simulink library "EngineSystemSubmodel"  (R2014b)
settings: Solver=ode45  StartTime=0.0  StopTime=10.0  FixedStep=1e-4  RelTol=1e-3
values from neighbouring files (symbols this model uses):
  D_turb_wheel = TC.TC_map.turb.D_wheel    [init_MVM.m]
  delta = 2    [Init8RTFLEX68D.m]    (also in Untitled2.m = fcn(p); fcn.m = zeros(size(p)))
  eta_turb_max = TC.TC_map.turb.eff_max    [init_MVM.m]
  flow_coeff_turb = [-1.585326540339;-4.823836967181;1.5853156139822]    [Init8RTFLEX68D.m]    (also in init_MVM.m = TC.TC_map.turb.flow_fit_coeff)
  fs = 0.0683    [Init8RTFLEX68D.m]    (also in NOxProcessGUI.m = varargin{2}; initHybrid.m; initMV.m; init_MVM.m = 0.0682925799315)
  genset = generators(1)    [runTempCyl4S.m]
  J_tc = TC.SAE_map_comp.inertia    [init_MVM.m]
  kai = 1.7    [Init8RTFLEX68D.m]
  Kb = 1*ones(engines,1)    [initHybrid.m]    (also in initMV.m; init_MVM.m = 1; init_ele.m = 1)
  Kd = 20*ones(engines,1)    [initHybrid.m]    (also in initMV.m; init_MVM.m = 10; init_ele.m = 20)
  Ki = 20*ones(engines,1)    [initHybrid.m]    (also in initMV.m; init_MVM.m = 10; init_ele.m = 20)
  Kp = 20*ones(engines,1)    [initHybrid.m]    (also in initMV.m; init_MVM.m = 10; init_ele.m = 20)
  Load_amp = x(4) + xRef(i)    [GetErrGensetResp.m]    (also in runsimulation.m = 0.55; runsimulationRecovery.m = InitialLoad(jj) + LoadStep(ii))
  Load_bias = x(4)    [GetErrGensetResp.m]    (also in runsimulation.m = 0.15; runsimulationRecovery.m = InitialLoad(jj))
  Load_index = 1    [GetErrGensetResp.m]    (also in runsimulation.m; runsimulationRecovery.m)
  N = x*noMol    [NOxProcessGUI.m]    (also in initHybrid.m = .1*ones(engines,1); initMV.m = .1*ones(engines,1); init_ele.m = 0.1)
  omegat0 = RPM_TC_initial/30*pi    [init_MVM.m]
  Start_time = 50    [GetErrGensetResp.m]    (also in runsimulation.m; runsimulationRecovery.m)
  T_load = 1    [GetErrGensetResp.m]    (also in runsimulation.m; runsimulationRecovery.m)
  T_ref_turb = TC.TC_map.turb.T_ref    [init_MVM.m]
  u0 = 0.2    [init_MVM.m]
  Uc_opt = TC.TC_map.turb.Uc_opt    [init_MVM.m]
  uMax = 1.5*ones(engines,1)    [initHybrid.m]    (also in initMV.m; init_MVM.m = 1.1; init_ele.m = 1.1)
  uMin = 0*ones(engines,1)    [initHybrid.m]    (also in initMV.m; init_MVM.m = 0.1; init_ele.m = 0.1)
undefined symbols (not defined in the file or in its folder): CAIPO, control, CV, cyl, eng, engSCont, omega0, rhoG0, Td, Ti, turbo, u_max, volDisp, vSCont, vSDes
undefined symbols (not defined in the file): comp_eff_map, comp_flow_map, n288_rep, npr, nsp, pr_rep, vComp
libraries: EngineSystemSubmodel x167, simulink x2
(part 1 of 5)
settings Model: Creator=yum  LastModifiedBy=yum

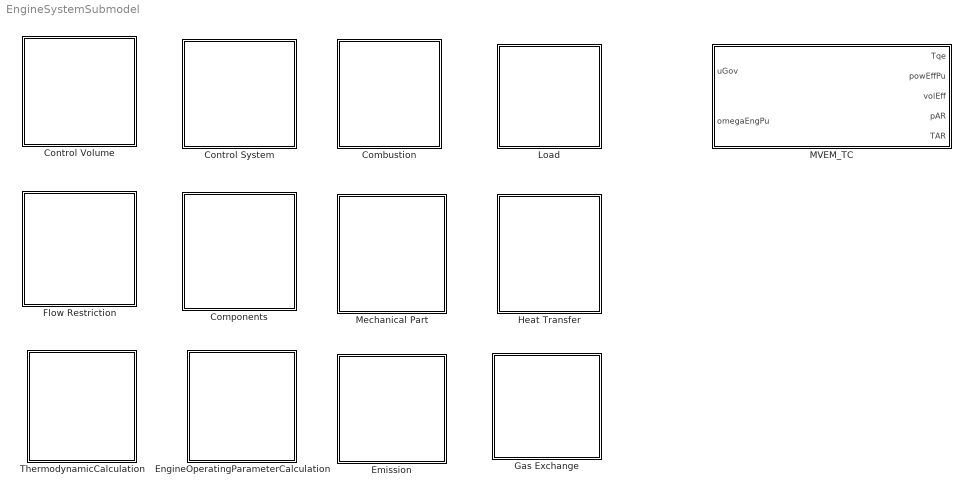
== system EngineSystemSubmodel ==
  Combustion : Subsystem
  Components : Subsystem
  Control System : Subsystem
  Control Volume : Subsystem
  Emission : Subsystem
  EngineOperatingParameterCalculation : Subsystem
  Flow Restriction : Subsystem
  Gas Exchange : Subsystem
  Heat Transfer : Subsystem
  Load : Subsystem
  MVEM_TC : Subsystem  mask{eng=genset.eng}
      mask prompts: eng "Genset parameters"
  Mechanical Part : Subsystem
  ThermodynamicCalculation : Subsystem

== system EngineSystemSubmodel/Combustion ==
  ROHR : Subsystem
  ROHRBus : Subsystem

== system EngineSystemSubmodel/Components ==
  ControlValve : Subsystem  mask{valveOpRef=0, KvRef=0}
      mask prompts: valveOpRef "Valve opening reference array (0~1)"; KvRef "Valve coefficient reference array (Kv) [m3/h]"
  EngCylinder2Stroke : Subsystem  mask{cylPar=eng.cyl, cylNo=1, cyl=0}
      mask prompts: cylPar "Cylinder parameters (struct)"; cylNo "Cylinder number"; cyl "Cylinder parameters"
      mask init:
      | cyl=cylPar(cylNo);
  EngCylinder2StrokeBus : Subsystem  mask{cylPar=eng.cyl, cylNo=1, cyl=0}
      mask prompts: cylPar "Engine Cylinder Parameters  (struct)"; cylNo "Cylinder number"; cyl "Engine Cylinder Parameters"
      mask init:
      | cyl=cylPar(cylNo);
  EngCylinder2StrokeBusConv : Subsystem  mask{cylPar=eng.cyl, cylNo=1, cyl=0}
      mask prompts: cylPar "Engine Cylinder Parameters  (struct)"; cylNo "Cylinder number"; cyl "Engine Cylinder Parameters"
      mask init:
      | cyl=cylPar(cylNo);
  EngCylinder2StrokeBusSSTune : Subsystem  mask{cylPar=eng.cyl, cylNo=1, cyl=eng.cyl}
      mask prompts: cylPar "Engine Cylinder Parameters  (struct)"; cylNo "Cylinder number"; cyl "Engine Cylinder Parameters"
      mask init:
      | cyl=cylPar(cylNo);
  EngCylinder2StrokeConv : Subsystem  mask{cylPar=eng.cyl, cylNo=1, cyl=0}
      mask prompts: cylPar "Cylinder Parameter (Struct)"; cylNo "Cylinder number"; cyl "Cylinder Parameter"
      mask init:
      | cyl = cylPar(cylNo);
  EngCylinder2StrokeSSTune : Subsystem  mask{cylPar=eng.cyl, cylNo=2, cyl=eng.cyl}
      mask prompts: cylPar "Cylinder parameters (struct)"; cylNo "Cylinder number"; cyl "Cylinder parameters"
      mask init:
      | cyl=cylPar(cylNo);
  EngCylinder2StrokeSSTune_ExtendedOutput : Subsystem  mask{cylPar=eng.cyl, cylNo=1, cyl=eng.cyl}
      mask prompts: cylPar "Cylinder Parameter (struct)"; cylNo "Cylinder number"; cyl "Cylinder Parameter"
      mask init:
      | cyl = cylPar(cylNo);
  EngCylinder2Stroke_ExtendedOutput : Subsystem  mask{cylPar=eng.cyl, cylNo=1, cyl=eng.cyl}
      mask prompts: cylPar "Cylinder Parameter (struct)"; cylNo "Cylinder number"; cyl "Cylinder Parameter"
      mask init:
      | cyl = cylPar(cylNo);
  EngCylinder2Zone2StrokeBusConv_Do Not Use : Subsystem  mask{cylPar=eng.cyl, cylNo=1, cyl=0}
      mask prompts: cylPar "Engine Cylinder Parameters  (struct)"; cylNo "Cylinder number"; cyl "Engine Cylinder Parameters"
      mask init:
      | cyl=cylPar(cylNo);
  EngCylinder2Zone2StrokeBus_Do Not Use : Subsystem  mask{cylPar=eng.cyl, cylNo=1, cyl=0}
      mask prompts: cylPar "Engine Cylinder Parameters  (struct)"; cylNo "Cylinder number"; cyl "Engine Cylinder Parameters"
      mask init:
      | cyl=cylPar(cylNo);
  EngCylinder4Stroke : Subsystem  mask{cyl=eng.cyl, cylNo=1}
      mask prompts: cyl "Engine Cylinder Parameters  (struct)"; cylNo "Cylinder number"
  EngineCylinderBlock2Stroke : Subsystem
  EngineCylinderBlock2StrokeBus : Subsystem
  EngineCylinderBlock2StrokeBusConv : Subsystem
  EngineCylinderBlock2StrokeBusSSTune : Subsystem
  EngineCylinderBlock2StrokeSSTune : Subsystem
  EngineCylinderBlock4StrokeBus : Subsystem
  ExhValve : Subsystem
  ExhValveBus : Subsystem
  ExhValveBusAEffAdjust : Subsystem
  InCylinderMV : Subsystem  mask{fs=0, Vd=0, LHV=0, Pe_nom=0, SFC=0, vol_eff_coeff1=0, vol_eff_coeff2=0, T_pe=0, nstroke=0, m_f_cyc_max=0, C1=0, p_a_inf=0, Pe0=0}
      mask prompts: fs "Stoichiometric fuel-air ratio"; Vd "Displacement volume (m3)"; LHV "Lower heating value of the fuel (J/kg)"; Pe_nom "Rated shaft power (W)"; SFC "Quadratic SFC curve coefficient (3x1)"; vol_eff_coeff1 "Volumetric efficiency coefficient for higher inlet pressure"; vol_eff_coeff2 "Volumetric efficiency coefficient for lower inlet pressure"; T_pe "Time constant for the torque development"; nstroke "Number of stroke"; m_f_cyc_max "Maximum amount of fuel injected per cycle (kg)"; C1 "Heat loss coefficient"; p_a_inf "Upper pressure limit for volumetric efficiency model 1 [bar]"; Pe0 "Initial power"
      mask TypeOptions fs: S-Function/fs
      mask TypeOptions Vd: S-Function/Vd
      mask TypeOptions LHV: S-Function/LHV
      mask TypeOptions Pe_nom: S-Function/Pe_nom
      mask TypeOptions SFC: S-Function/SFC
      mask TypeOptions vol_eff_coeff1: S-Function/vol_eff_coeff1
      mask TypeOptions vol_eff_coeff2: S-Function/vol_eff_coeff2
      mask TypeOptions T_pe: S-Function/T_pe
      mask TypeOptions nstroke: S-Function/nstroke
      mask TypeOptions m_f_cyc_max: S-Function/m_f_cyc_max
      mask TypeOptions C1: S-Function/C1
      mask TypeOptions p_a_inf: S-Function/p_a_inf
      mask TypeOptions Pe0: S-Function/Pe0
  InCylinderMVBus : Subsystem  mask{cyl=eng.cyl}
  IntakePort : Subsystem
  IntakePortBus : Subsystem
  IntakeValve : Subsystem
  IntakeValveBus : Subsystem
  IntakeValveBusAEffAdjust : Subsystem
  Turbocharger : Subsystem  mask{turbo=turbo}
      mask prompts: turbo "Turbocharger parameters struct"
  TurbochargerFullModel : Subsystem  mask{turbo=eng.turbo}
      mask prompts: turbo "Turbocharger parameters"
  TurbochargerMV : Subsystem  mask{fs=fs, J_tc=J_tc, omegat0=omegat0, comp_flow_map=comp_flow_map, comp_eff_map=comp_eff_map, pr_rep=pr_rep, n_288_rep=n288_rep, npr=npr, nsp=nsp, flow_coeff_turb=flow_coeff_turb, D_wheel_turb=D_turb_wheel, Uc_opt=Uc_opt, eta_turb_max=eta_turb_max, T_ref=T_ref_turb}
      mask prompts: fs "Stoichiometric fuel-air ratio"; J_tc "Mass moment of inertia of a rotor"; omegat0 "Initial rotor speed"; comp_flow_map "Compressor map for corrected flow"; comp_eff_map "Compressor map for efficiency"; pr_rep "Pressure ratio arry for look-up in compressor map"; n_288_rep "Corrected speed array for look-up in compressor map"; npr "Length of pressure ratio array for look-up in compressor map"; nsp "Length of corrected speed array for look-up in compressor map"; flow_coeff_turb "Flow coefficient for turbine model"; D_wheel_turb "Turbine wheel diameter"; Uc_opt "Optimal blade speed ratio"; eta_turb_max "Maximum efficiency"; T_ref "Reference temperature for turbine flow"
  WasteGate : Subsystem

== system EngineSystemSubmodel/Control System ==
  ECSParamId : Subsystem  mask{control=eng.control}
      mask prompts: control "Control Parameters"
  ECSTrans : Subsystem  mask{control=eng.control}
      mask prompts: control "Engine Control Parameters"
  ECSTrans1 : Subsystem  mask{control=eng.control}
      mask prompts: control "Engine Control Parameters"
  ECSTransSmokeLim : Subsystem  mask{control=eng.control}
      mask prompts: control "Engine Control Parameters"
  Governor : Subsystem
  Governor_SpeedControl : Subsystem  mask{Kp=Kp, Kd=Kd, N=0, Ki=Ki, Kb=Kb, omega0=omega0, u_min=u_max, u_max=u_max, u0=u0}
      mask prompts: Kp "Proportional gain"; Kd "Differential gain"; N "Dirty derivative gain"; Ki "Integral gain"; Kb "Back-calculation gain"; omega0 "Initial engine speed [pu]"; u_min "Minimum governor output"; u_max "Maximum governor output"; u0 "Initial governor output"
      mask TypeOptions Kp: PID controller/Kp
      mask TypeOptions Kd: PID controller/Kd
      mask TypeOptions N: PID controller/N
      mask TypeOptions Ki: PID controller/Ki
      mask TypeOptions Kb: PID controller/Kb
      mask TypeOptions omega0: PID controller/omega0
      mask TypeOptions u_min: PID controller/u_min
      mask TypeOptions u_max: PID controller/u_max
      mask TypeOptions u0: PID controller/u0
  LPFilterBW4 : S-Function  FunctionName=lowPassFilterBW4  Parameters=BW,y0  EnableBusSupport=off  mask{BW=0, y0=0}
      mask prompts: BW "Bandwidth [Hz]"; y0 "Initial output"
  PIDControlAntiWinding : Subsystem  mask{Kp=Kp, Td=Td, N=N, Ti=Ti, uMax=uMax, uMin=uMin, u0=u0, Kb=Kb}
      mask prompts: Kp "Proportional gain"; Td "Time constant for derivative term"; N "Gain for dirty derivative"; Ti "Time constant for integral term"; uMax "Maximum output"; uMin "Minimum output"; u0 "Initial output"; Kb "Back propagation gain"
  Smoke Limiter : Subsystem
  Smoke Limiter MV : Subsystem  mask{fs=genset.eng.fs, Vd=genset.eng.vD, F_max=genset.eng.fMax, m_f_cyc_max=genset.eng.mFCycMax}
      mask prompts: fs "Stoichiometric fuel-air ratio"; Vd "Displacement volume (m3)"; F_max "Maximum fuel-air equivalent ratio"; m_f_cyc_max "Maximum fuel injection @ rated power (kg)"
  SpeedController : Subsystem  mask(20-sim 4.4 S-Function block){Kp=control.speed.Kp, Td=control.speed.Td, N=control.speed.N, Ti=control.speed.Ti, max=control.speed.uMax, min=control.speed.uMin, u0=control.speed.u0}
      mask prompts: Kp "Proportional gain"; Td "Time constant for derivative term (s)"; N "Derivative filter coefficient"; Ti "Time constant for integral term"; max "Maximum output"; min "Minimum output"; u0 "Initial output"
      mask help:
      | This block is generated by the 20-sim ANSI-C Code Generator.
      |
      | * look under the mask to get information on the ports
      | * press Help for more detailed information
      | * the parameters of this block are:
      mask Help:
      | This block is generated by the 20-sim ANSI-C Code Generator<br>
      | The block parameters are:<br><blockquote></blockquote>
      | Generated at:<br>
      | <blockquote><b>date:  </b>August 27, 2014<br>
      | <b>time:  </b>10:21:01 pm<br></blockquote>
      | From the following 20-sim model:<br>
      | <blockquote><b>submodel:  </b>SpeedController<br>
      | <b>model:  </b>8RT-FLEX68-D_transient<br>
      | <b>file:  </b>E:\DBox\Dropbox\Study\Research Project\SHI Project\Program\BG\8RT-FLEX68-D_transient.emx<br>
      | <b>experiment:  </b>E:\DBox\Dropbox\Study\Research Project\SHI Project\Program\BG\8RT-FLEX68-D_transient.emx<br></blockquote>
      | Using the following 20-sim license:<br>
      | <blockquote><b>user:  </b>Norwegian University of Science and Technology <br>
      | <b>from:  </b>20-sim 4.4 Student License<br>
      | <b>build: </b>4.4.1.4356<br></blockquote>

== system EngineSystemSubmodel/Control Volume ==
  ThdynCV2ZoneBG_VarVolBus : Subsystem  mask{CV=cyl.init}
      mask prompts: CV "Name of the control volume"
  ThdynCV2ZoneConv_VarVolBus : Subsystem  mask{CV=cyl.init}
      mask prompts: CV "Name of the control volume"
  ThdynCVConv_VarVol : Subsystem  mask{CV=CV}
      mask prompts: CV "Name of the control volume"
  ThdynCVConv_VarVolBus : Subsystem  mask{CV=CV}
      mask prompts: CV "Name of the control volume"
  ThdynCV_FixVol : Subsystem  mask{CV=CV}
      mask prompts: CV "Name of the control volume"
  ThdynCV_VarVol : Subsystem  mask{CV=CV}
      mask prompts: CV "Name of the control volume"
  ThdynCV_VarVolBus : Subsystem  mask{CV=CV}
      mask prompts: CV "Name of control volume"

== system EngineSystemSubmodel/Emission ==
  NOx : Subsystem

== system EngineSystemSubmodel/EngineOperatingParameterCalculation ==
  SFCCyc : Subsystem
  pCompCalc : Subsystem  mask{vComp=vComp}
      mask prompts: vComp "Compression volume"
  pMaxFinder : Subsystem
  resetCyc : Subsystem
  volEffCalc : Subsystem  mask{RPMMax=eng.RPMMax, nStroke=eng.nStroke}
      mask prompts: RPMMax "Maximum engine speed"; nStroke "Number of stroke"
  workPerCycle : Subsystem

== system EngineSystemSubmodel/Flow Restriction ==
  AirWaterCooler : Subsystem  mask{cAC=eng.cAC}
      mask prompts: cAC "Charge Air Cooler Parameter"
  AirWaterCoolerBus : Subsystem
  Compressor : Subsystem  mask{comp=turbo.comp}
      mask prompts: comp "Compressor parameters"
  CompressorBus : Subsystem
  CompressorFullMap : Subsystem  mask{comp=turbo.comp}
      mask prompts: comp "Compressor Parameters"
  IdealNozzle : Subsystem
  IdealNozzleBus : Subsystem
  Turbine : Subsystem  mask{turb=turbo.turb}
      mask prompts: turb "Turbine Parameters"
  TurbineBus : Subsystem
  TurbineFullMap : Subsystem  mask{turb=turbo.turb}
      mask prompts: turb "Turbine parameters"
  TurbineMV : Subsystem  mask{fs=0, flow_coeff_turb=0, D_turb_wheel=0, Uc_opt=0, eta_turb_max=0}
      mask prompts: fs "Stoichiometric fuel-air ratio"; flow_coeff_turb "Flow coefficient for turbine model (3x1)"; D_turb_wheel "Turbine wheel diameter (m)"; Uc_opt "Optimal blade speed ratio"; eta_turb_max "Maximum efficiency"
  TurbineMVBus : Subsystem
  blower : Subsystem  mask{blower=eng.blower}
      mask prompts: blower "Blower Parameter Struct"
  blowerFit : Subsystem

== system EngineSystemSubmodel/Gas Exchange ==
  Scavenging : Subsystem
  ScavengingBus : Subsystem

== system EngineSystemSubmodel/Heat Transfer ==
  EngCylHeatTransfer : Subsystem
  EngCylHeatTransferBus : Subsystem
  EngCylHeatTransferSSTune : Subsystem
  EngCylHeatTransferSSTuneBus : Subsystem

== system EngineSystemSubmodel/Load ==
  Load : Subsystem  mask{Load_index=Load_index, Load_amp=Load_amp, Load_bias=Load_bias, Start_time=Start_time, T_load=T_load}
      mask prompts: Load_index "Load index"; Load_amp "Load amplitude"; Load_bias "Load in bias"; Start_time "Load initiation time"; T_load "Period of the load"
      mask help:
      | Load Selection and Definition
      | Load_index   Load_amp   Load_bias   Start_time    T_load
      | 1-Step,             Final,      Initial,        Step time,      N/A,
      | 2-Sine,             amp,        bias,           Delay,          Period
      | 3-Ramp,             Slope,      Initial,        Start time,     N/A
      | 4-User input        N/A,        Initial,        Delay,          N/A
      | 5-External input    N/A,        Initial,        Delay,          N/A
      | 6-Constant          N/A,        Load,           N/A,            N/A
  Propeller : MATLAB Function  TreatAsAtomicUnit=on

== system EngineSystemSubmodel/MVEM_TC ==
  uGov : Inport
  omegaEngPu : Inport  Port=2
  AirWaterCoolerNV : EngineSystemSubmodel/Flow Restriction/AirWaterCoolerBus
  Bus Creator : BusCreator  Inputs=3
  Bus Creator1 : BusCreator  Inputs=3
  Bus Selector : BusSelector  OutputSignals=p,T
  Bus Selector1 : BusSelector  OutputSignals=dmd,dEd,dmbd
  Bus Selector2 : BusSelector  OutputSignals=dmu,dEu,dmbu
  Bus Selector3 : BusSelector  OutputSignals=dmu,dEu,dmbu
  Bus Selector4 : BusSelector  OutputSignals=dmd,dEd,dmbd
  Bus Selector6 : BusSelector  OutputSignals=dmd,dEd,dmbd
  Bus Selector8 : BusSelector  OutputSignals=dmu,dEu,dmbu
  CompressorNV : EngineSystemSubmodel/Flow Restriction/CompressorBus
  Constant : Constant  Value=genset.eng.pAmb
  Constant1 : Constant  Value=0
  Constant2 : Constant  Value=0
  Constant3 : Constant  Value=genset.eng.tCW
  Constant4 : Constant  Value=0
  Constant5 : Constant  Value=genset.eng.tAmb
  Constant8 : Constant  Value=genset.eng.fAmb
  Constant9 : Constant  Value=genset.eng.pBack
  Gain : Gain  Gain=genset.eng.omegaENom
  Gain1 : Gain  Gain=1/genset.eng.tqShaftNom
  InCylinderMV1 : EngineSystemSubmodel/Components/InCylinderMVBus  cyl=eng.cyl
  Sum{,1..8} (9 alike) : Sum  Inputs=-+|
  Terminator{,1..4} (5 alike) : Terminator
  TurbineMV1 : EngineSystemSubmodel/Flow Restriction/TurbineMVBus
  TurbochargerShaft : Subsystem
  airReceiver : EngineSystemSubmodel/Control Volume/ThdynCV_VarVolBus  CV=CV
  exhaustReceiver : EngineSystemSubmodel/Control Volume/ThdynCV_VarVolBus  CV=CV
  pipe : EngineSystemSubmodel/Control Volume/ThdynCV_VarVolBus  CV=CV
  Tqe : Outport
  powEffPu : Outport  Port=2
  volEff : Outport  Port=3
  pAR : Outport  Port=4
  TAR : Outport  Port=5
  wires:
  TurbochargerShaft/1(omegaTC) -> [omegaT], CompressorNV/3  "omegaTC"
  [turbTq] -> TurbochargerShaft/2(tqTurb)  "tqTurb"
  CompressorNV/3 -> TurbochargerShaft/1(tqComp)  "tqComp"
  InCylinderMV1/3 -> Gain1/1
  CompressorNV/1 -> Terminator4/1
  CompressorNV/4 -> Terminator3/1
  Bus Selector/2 -> TAR/1  "<T>"
  Bus Selector/1 -> pAR/1  "<p>"
  Gain1/1 -> Tqe/1
  uGov/1 -> InCylinderMV1/4
  InCylinderMV1/4 -> volEff/1
  Constant3/1 -> AirWaterCoolerNV/3
  CompressorNV/2 -> Bus Selector1/1
  Bus Selector4/1 -> Sum3/2  "<dmd>"
  Constant1/1 -> airReceiver/4
  Bus Selector4/3 -> Sum5/2  "<dmbd>"
  Bus Selector6/3 -> Sum2/2  "<dmbd>"
  InCylinderMV1/2 -> Bus Selector4/1
  Sum4/1 -> exhaustReceiver/2
  Bus Selector4/2 -> Sum4/2  "<dEd>"
  Sum2/1 -> airReceiver/3
  Sum1/1 -> airReceiver/2
  Sum5/1 -> exhaustReceiver/3
  Constant2/1 -> exhaustReceiver/4
  Sum3/1 -> exhaustReceiver/1  "dm"
  Bus Selector6/2 -> Sum1/2  "<dEd>"
  Bus Selector6/1 -> Sum/2  "<dmd>"
  AirWaterCoolerNV/1 -> Bus Selector8/1
  Bus Selector8/3 -> Sum8/1  "<dmbu>"
  pipe/1 -> AirWaterCoolerNV/1, CompressorNV/2
  Sum8/1 -> pipe/3
  Gain/1 -> InCylinderMV1/3
  Bus Selector8/1 -> Sum6/1  "<dmu>"
  Sum7/1 -> pipe/2
  Bus Selector8/2 -> Sum7/1  "<dEu>"
  AirWaterCoolerNV/2 -> Bus Selector6/1
  Sum6/1 -> pipe/1  "dm"
  InCylinderMV1/5 -> powEffPu/1
  TurbineMV1/1 -> Bus Selector3/1
  [omegaT] -> TurbineMV1/3
  Bus Selector3/1 -> Sum3/1  "<dmu>"
  Bus Creator/1 -> [pTFBComp]
  Bus Selector1/1 -> Sum6/2  "<dmd>"
  Bus Selector1/3 -> Sum8/2  "<dmbd>"
  Bus Selector1/2 -> Sum7/2  "<dEd>"
  Constant4/1 -> pipe/4
  airReceiver/1 -> AirWaterCoolerNV/2, Bus Selector/1, InCylinderMV1/1
  omegaEngPu/1 -> Gain/1
  exhaustReceiver/1 -> InCylinderMV1/2, TurbineMV1/1
  Bus Selector2/3 -> Sum2/1  "<dmbu>"
  Bus Selector2/2 -> Sum1/1  "<dEu>"
  Sum/1 -> airReceiver/1  "dm"
  Bus Selector2/1 -> Sum/1  "<dmu>"
  InCylinderMV1/1 -> Bus Selector2/1
  Bus Selector3/3 -> Sum5/1  "<dmbu>"
  TurbineMV1/3 -> [turbTq]
  [pTFATurb] -> TurbineMV1/2
  [pTFBComp] -> CompressorNV/1
  Bus Selector3/2 -> Sum4/1  "<dEu>"
  Constant9/1 -> Bus Creator1/1  "p"
  Bus Creator1/1 -> [pTFATurb]
  Constant/1 -> Bus Creator/1  "p"
  Constant8/1 -> Bus Creator/3, Bus Creator1/3  "F"
  Constant5/1 -> Bus Creator/2, Bus Creator1/2  "T"
  TurbineMV1/5 -> Terminator1/1
  TurbineMV1/4 -> Terminator2/1
  TurbineMV1/2 -> Terminator/1

== system EngineSystemSubmodel/Mechanical Part ==
  CrankMechKinematic : Subsystem
  Shaft : Subsystem

== system EngineSystemSubmodel/ThermodynamicCalculation ==
  GetXCombGas : Subsystem
  ThdynCombGasZach : Subsystem

== system EngineSystemSubmodel/Combustion/ROHR ==
  pTF : Inport
  u_gov : Inport  Port=2
  phiInj : Inport  Port=3
  phi : Inport  Port=4
  omega : Inport  Port=5
  Demux : Demux  Outputs=3
  S-Function : S-Function  FunctionName=combState  Parameters=cyl.comb.mqfCycMax,cyl.comb.wiebePara,eng.nStroke  EnableBusSupport=off
  S-Function1 : S-Function  FunctionName=CombWiebe  Parameters=eng.hn, cyl.comb.wiebePara  EnableBusSupport=off
  Terminator : Terminator
  dmEmb : Outport
  combState : Outport  Port=2
  phiIg : Outport  Port=3
  mqf : Outport  Port=4
  wires:
  S-Function/4 -> mqf/1, S-Function1/4  "mqf"
  S-Function/3 -> phiIg/1, S-Function1/3  "phiIg"
  S-Function/2 -> S-Function1/2  "phiComb"
  S-Function/1 -> S-Function1/1, combState/1  "combState"
  S-Function1/1 -> dmEmb/1
  Demux/3 -> Terminator/1
  Demux/2 -> S-Function/6  "T"
  Demux/1 -> S-Function/5  "p"
  pTF/1 -> Demux/1
  omega/1 -> S-Function/4, S-Function1/5
  u_gov/1 -> S-Function/3
  phiInj/1 -> S-Function/2
  phi/1 -> S-Function/1

== system EngineSystemSubmodel/Combustion/ROHRBus ==
  pTF : Inport
  u_gov : Inport  Port=2
  phiInj : Inport  Port=3
  phi : Inport  Port=4
  omega : Inport  Port=5
  Bus Creator : BusCreator  Inputs=3
  Bus Selector : BusSelector  OutputSignals=p,T
  Demux1 : Demux  Outputs=3
  S-Function : S-Function  FunctionName=combState  Parameters=cyl.comb.mqfCycMax,cyl.comb.wiebePara,eng.nStroke  EnableBusSupport=off
  S-Function1 : S-Function  FunctionName=CombWiebe  Parameters=eng.hn, cyl.comb.wiebePara  EnableBusSupport=off
  dmEmb : Outport
  combState : Outport  Port=2
  phiIg : Outport  Port=3
  mqf : Outport  Port=4
  wires:
  S-Function/4 -> mqf/1, S-Function1/4  "mqf"
  S-Function/3 -> phiIg/1, S-Function1/3  "phiIg"
  S-Function/2 -> S-Function1/2  "phiComb"
  S-Function/1 -> S-Function1/1, combState/1  "combState"
  S-Function1/1 -> Demux1/1
  pTF/1 -> Bus Selector/1
  omega/1 -> S-Function/4, S-Function1/5
  u_gov/1 -> S-Function/3
  phiInj/1 -> S-Function/2
  phi/1 -> S-Function/1
  Demux1/2 -> Bus Creator/2  "dE"
  Demux1/3 -> Bus Creator/3  "dmb"
  Demux1/1 -> Bus Creator/1  "dm"
  Bus Selector/2 -> S-Function/6  "<T>"
  Bus Selector/1 -> S-Function/5  "<p>"
  Bus Creator/1 -> dmEmb/1

== system EngineSystemSubmodel/Components/ControlValve ==
  pTFu : Inport
  pTFd : Inport  Port=2
  u : Inport  Port=3
  Bus Creator : BusCreator  Inputs=3
  Bus Selector : BusSelector  OutputSignals=p,T
  Bus Selector1 : BusSelector  OutputSignals=p
  Bus Selector2 : BusSelector  OutputSignals=p,T,F  OutputAsBus=on
  Bus Selector3 : BusSelector  OutputSignals=h
  Bus Selector4 : BusSelector  OutputSignals=F
  Constant : Constant  Value=eng.fs
  Constant1 : Constant
  Gain : Gain  Gain=rhoG0
  Gain1 : Gain  Gain=519
  Gain2 : Gain  Gain=1/3600
  Gain3 : Gain  Gain=1e-5
  Gain4 : Gain  Gain=1e-5
  MATLAB Function : MATLAB Function  TreatAsAtomicUnit=on  mask{x=valveOpRef, y=KvRef}
      mask prompts: x "Valve opening reference array"; y "Valve flow coefficient reference array (Kv) [m3/h]"
  Product{,2..4} (4 alike) : Product
  Product1 : Product  Inputs=*/
  Product5 : Product  Inputs=*/*
  Sqrt : Sqrt  SaturateOnIntegerOverflow=on
  Sum : Sum  Inputs=|+-
  Sum1 : Sum  Inputs=|++
  ThdynCombGasZach : EngineSystemSubmodel/ThermodynamicCalculation/ThdynCombGasZach
  Out1 : Outport
  wires:
  pTFd/1 -> Bus Selector1/1
  Bus Selector1/1 -> Gain4/1  "<p>"
  Sum/1 -> Product/1
  Product/1 -> Gain/1
  Gain/1 -> Product1/1
  Bus Selector/2 -> Product1/2  "<T>"
  Product1/1 -> Sqrt/1
  Sqrt/1 -> Gain1/1
  u/1 -> MATLAB Function/1(u)
  Gain1/1 -> Product2/1
  MATLAB Function/1(y1) -> Gain2/1
  Bus Selector2/1 -> ThdynCombGasZach/1
  ThdynCombGasZach/1 -> Bus Selector3/1
  Bus Selector3/1 -> Product3/1  "<h>"
  Product2/1 -> Product5/3, Product3/2, Bus Creator/1  "dmu"
  Product3/1 -> Bus Creator/2  "dEu"
  Constant/1 -> Product4/1
  pTFu/1 -> Bus Selector4/1, Bus Selector2/1, Bus Selector/1
  Bus Selector4/1 -> Product4/2  "<F>"
  Product4/1 -> Product5/1, Sum1/1  "fsF"
  Constant1/1 -> Sum1/2
  Sum1/1 -> Product5/2
  Product5/1 -> Bus Creator/3  "dmbu"
  Bus Creator/1 -> Out1/1
  Gain2/1 -> Product2/2
  Bus Selector/1 -> Gain3/1  "<p>"
  Gain3/1 -> Sum/1
  Gain4/1 -> Sum/2, Product/2

== system EngineSystemSubmodel/Components/EngCylinder2Stroke ==
  uGov : Inport
  phiInj : Inport  Port=2
  cAStartNom : Inport  Port=3
  dCALiftUp : Inport  Port=4
  pTF_u : Inport  Port=5
  pTF_d : Inport  Port=6
  omega : Inport  Port=7
  Constant : Constant  Value=0
  CrankMechKinematic : EngineSystemSubmodel/Mechanical Part/CrankMechKinematic
  Demux{,1..3,5} (5 alike) : Demux  Outputs=3
  EngCylHeatTransfer : EngineSystemSubmodel/Heat Transfer/EngCylHeatTransfer
  ExhValve : EngineSystemSubmodel/Components/ExhValve
  IntakePort1 : EngineSystemSubmodel/Components/IntakePort
  Mux : Mux  Inputs=3
  Mux1 : Mux  Inputs=3
  Mux2 : Mux  Inputs=2
  Mux3 : Mux  Inputs=3
  ROHR1 : EngineSystemSubmodel/Combustion/ROHR
  Scavenging : EngineSystemSubmodel/Gas Exchange/Scavenging
  Sum : Sum  Inputs=++--
  Sum1 : Sum  Inputs=++|
  Terminator{1..3,6..9,11,13..14,16} (11 alike) : Terminator
  ThdynCV_VarVol1 : EngineSystemSubmodel/Control Volume/ThdynCV_VarVol  CV=cyl.init
  pCyl : Outport
  phi : Outport  Port=2
  teampWall : Outport  Port=3
  phiIg : Outport  Port=4
  dQ : Outport  Port=5
  dmEmb_u : Outport  Port=6
  dmEmb_d : Outport  Port=7
  Tq : Outport  Port=8
  dmb : Outport  Port=9
  wires:
  Mux3/1 -> ExhValve/4
  [cAStartNom] -> ExhValve/2
  dCALiftUp/1 -> [dCALiftUp]
  cAStartNom/1 -> [cAStartNom]
  ExhValve/2 -> dmEmb_d/1
  Mux2/1 -> Terminator2/1
  ExhValve/4 -> Mux2/2
  ExhValve/3 -> Mux2/1
  Mux1/1 -> Terminator1/1
  IntakePort1/5 -> Mux1/3
  IntakePort1/4 -> Mux1/2
  IntakePort1/3 -> Mux1/1
  ROHR1/3 -> phiIg/1  "phiIg"
  EngCylHeatTransfer/2 -> teampWall/1
  Demux/3 -> Terminator7/1
  Demux/2 -> Terminator6/1
  Constant/1 -> Mux/3, Mux/1
  Mux/1 -> Sum/4
  Sum1/1 -> Mux/2
  EngCylHeatTransfer/1 -> Sum1/1, dQ/1
  ThdynCV_VarVol1/3 -> EngCylHeatTransfer/2  "vCyl"
  IntakePort1/1 -> dmEmb_u/1
  omega/1 -> ROHR1/5, EngCylHeatTransfer/3, CrankMechKinematic/2
  phiInj/1 -> ROHR1/3
  CrankMechKinematic/2 -> Tq/1
  Demux/1 -> CrankMechKinematic/3
  CrankMechKinematic/3 -> Sum1/2
  uGov/1 -> ROHR1/2
  CrankMechKinematic/1 -> ThdynCV_VarVol1/2
  ThdynCV_VarVol1/2 -> CrankMechKinematic/1, pCyl/1
  ThdynCV_VarVol1/1 -> EngCylHeatTransfer/1, Demux2/1, IntakePort1/3, ROHR1/1  "pTFCyl"
  Sum/1 -> ThdynCV_VarVol1/1
  ExhValve/1 -> Sum/3
  ROHR1/1 -> Sum/2, Demux1/1  "dmEmbComb"
  Demux1/1 -> dmb/1
  Demux1/2 -> Terminator8/1
  Demux1/3 -> Terminator9/1
  ROHR1/4 -> Terminator3/1
  pTF_u/1 -> [pTFIn], Demux/1, IntakePort1/2
  pTF_d/1 -> ExhValve/5
  ROHR1/2 -> [combState]
  [pTFIn] -> Demux3/1
  Demux3/1 -> Scavenging/4  "pIn"
  Demux3/2 -> Scavenging/5
  Demux3/3 -> Scavenging/6
  [mDotIn] -> Scavenging/7
  CrankMechKinematic/4 -> [phi], IntakePort1/1, phi/1, Scavenging/9, ExhValve/1
  IntakePort1/2 -> Demux5/1, Sum/1
  Demux5/2 -> Terminator11/1
  Demux5/3 -> Terminator16/1
  Demux5/1 -> [mDotIn]
  [combState] -> Scavenging/8
  [phi] -> ROHR1/4
  Scavenging/3 -> Terminator13/1
  Scavenging/4 -> Terminator14/1
  Demux2/2 -> Scavenging/2
  Demux2/1 -> Mux3/1, Scavenging/1
  Demux2/3 -> Scavenging/3
  Scavenging/1 -> Mux3/2  "TOut"
  Scavenging/2 -> Mux3/3  "FOut"
  [dCALiftUp] -> ExhValve/3

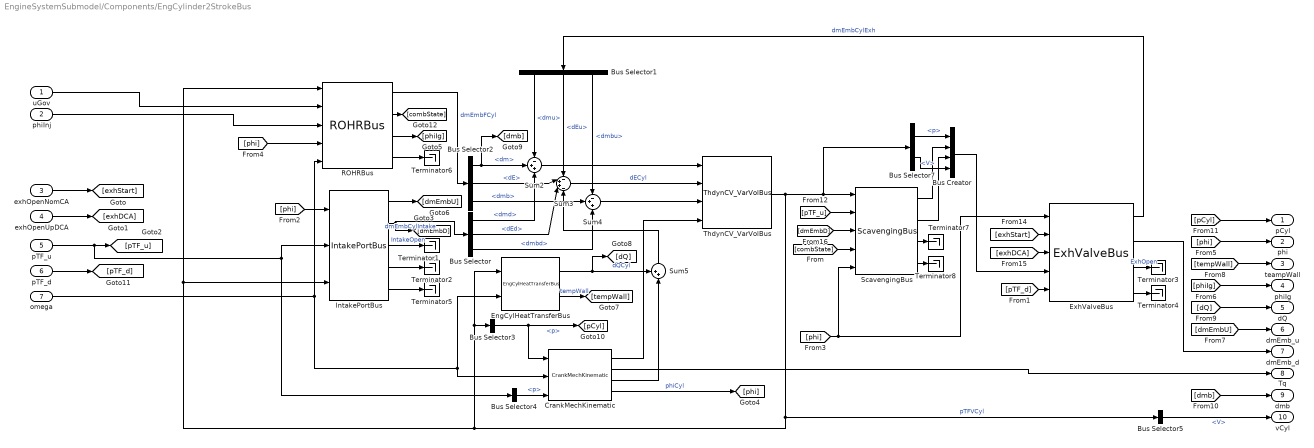
== system EngineSystemSubmodel/Components/EngCylinder2StrokeBus ==
  uGov : Inport
  phiInj : Inport  Port=2
  exhOpenNomCA : Inport  Port=3
  exhOpenUpDCA : Inport  Port=4
  pTF_u : Inport  Port=5
  pTF_d : Inport  Port=6
  omega : Inport  Port=7
  Bus Creator : BusCreator
  Bus Selector : BusSelector  OutputSignals=dmd,dEd,dmbd
  Bus Selector1 : BusSelector  OutputSignals=dmu,dEu,dmbu
  Bus Selector2 : BusSelector  OutputSignals=dm,dE,dmb
  Bus Selector3 : BusSelector  OutputSignals=p
  Bus Selector4 : BusSelector  OutputSignals=p
  Bus Selector5 : BusSelector  OutputSignals=V
  Bus Selector7 : BusSelector  OutputSignals=p,V
  CrankMechKinematic : EngineSystemSubmodel/Mechanical Part/CrankMechKinematic
  EngCylHeatTransferBus : EngineSystemSubmodel/Heat Transfer/EngCylHeatTransferBus
  ExhValveBus : EngineSystemSubmodel/Components/ExhValveBus
  IntakePortBus : EngineSystemSubmodel/Components/IntakePortBus
  ROHRBus : EngineSystemSubmodel/Combustion/ROHRBus
  ScavengingBus : EngineSystemSubmodel/Gas Exchange/ScavengingBus
  Sum2 : Sum  Inputs=-++
  Sum3 : Sum  Inputs=-++-
  Sum4 : Sum  Inputs=-++
  Sum5 : Sum  Inputs=++|
  Terminator{1..8} (8 alike) : Terminator
  ThdynCV_VarVolBus : EngineSystemSubmodel/Control Volume/ThdynCV_VarVolBus  CV=cyl.init
  pCyl : Outport
  phi : Outport  Port=2
  teampWall : Outport  Port=3
  phiIg : Outport  Port=4
  dQ : Outport  Port=5
  dmEmb_u : Outport  Port=6
  dmEmb_d : Outport  Port=7
  Tq : Outport  Port=8
  dmb : Outport  Port=9
  vCyl : Outport  Port=10
  wires:
  IntakePortBus/2 -> [dmEmbD], Bus Selector/1  "dmEmbCylIntake"
  Sum2/1 -> ThdynCV_VarVolBus/1
  Sum3/1 -> ThdynCV_VarVolBus/2  "dECyl"
  Sum4/1 -> ThdynCV_VarVolBus/3
  ExhValveBus/1 -> Bus Selector1/1  "dmEmbCylExh"
  Bus Selector1/1 -> Sum2/1  "<dmu>"
  Bus Selector1/2 -> Sum3/1  "<dEu>"
  Bus Selector1/3 -> Sum4/1  "<dmbu>"
  Bus Selector/1 -> Sum2/3  "<dmd>"
  ROHRBus/1 -> Bus Selector2/1  "dmEmbFCyl"
  Bus Selector2/1 -> [dmb], Sum2/2  "<dm>"
  Bus Selector/2 -> Sum3/3  "<dEd>"
  Bus Selector/3 -> Sum4/3  "<dmbd>"
  Bus Selector2/3 -> Sum4/2  "<dmb>"
  omega/1 -> ROHRBus/5, CrankMechKinematic/2, EngCylHeatTransferBus/2
  Bus Selector3/1 -> CrankMechKinematic/1, [pCyl]  "<p>"
  CrankMechKinematic/2 -> Tq/1
  CrankMechKinematic/1 -> ThdynCV_VarVolBus/4
  EngCylHeatTransferBus/1 -> [dQ], Sum5/1  "dQCyl"
  CrankMechKinematic/4 -> [phi]  "phiCyl"
  [phi] -> IntakePortBus/1
  [phi] -> ExhValveBus/1, ScavengingBus/5
  pTF_u/1 -> [pTF_u], IntakePortBus/2, Bus Selector4/1
  Bus Selector4/1 -> CrankMechKinematic/3  "<p>"
  exhOpenNomCA/1 -> [exhStart]
  exhOpenUpDCA/1 -> [exhDCA]
  [phi] -> ROHRBus/4
  ROHRBus/3 -> [phiIg]
  [phiIg] -> phiIg/1
  [phi] -> phi/1
  IntakePortBus/1 -> [dmEmbU]
  [dmEmbU] -> dmEmb_u/1
  ExhValveBus/2 -> dmEmb_d/1
  EngCylHeatTransferBus/2 -> [tempWall]  "tempWall"
  [tempWall] -> teampWall/1
  [dQ] -> dQ/1
  [dmb] -> dmb/1
  [pCyl] -> pCyl/1
  [exhStart] -> ExhValveBus/2
  [exhDCA] -> ExhValveBus/3
  ROHRBus/2 -> [combState]
  IntakePortBus/3 -> Terminator1/1  "IntakeOpen"
  IntakePortBus/4 -> Terminator2/1
  ExhValveBus/3 -> Terminator3/1  "ExhOpen"
  ExhValveBus/4 -> Terminator4/1
  Sum5/1 -> Sum3/4
  Bus Selector2/2 -> Sum3/2  "<dE>"
  uGov/1 -> ROHRBus/2
  phiInj/1 -> ROHRBus/3
  pTF_d/1 -> [pTF_d]
  [pTF_d] -> ExhValveBus/5
  CrankMechKinematic/3 -> Sum5/2
  IntakePortBus/5 -> Terminator5/1
  Bus Selector5/1 -> vCyl/1  "<V>"
  ROHRBus/4 -> Terminator6/1
  [pTF_u] -> ScavengingBus/2
  [dmEmbD] -> ScavengingBus/3
  [combState] -> ScavengingBus/4
  ScavengingBus/3 -> Terminator7/1
  ScavengingBus/4 -> Terminator8/1
  ThdynCV_VarVolBus/1 -> Bus Selector7/1, ScavengingBus/1, ROHRBus/1, IntakePortBus/3, EngCylHeatTransferBus/1, Bus Selector3/1, Bus Selector5/1  "pTFVCyl"
  Bus Selector7/1 -> Bus Creator/1  "<p>"
  Bus Creator/1 -> ExhValveBus/4
  ScavengingBus/1 -> Bus Creator/2
  ScavengingBus/2 -> Bus Creator/3
  Bus Selector7/2 -> Bus Creator/4  "<V>"

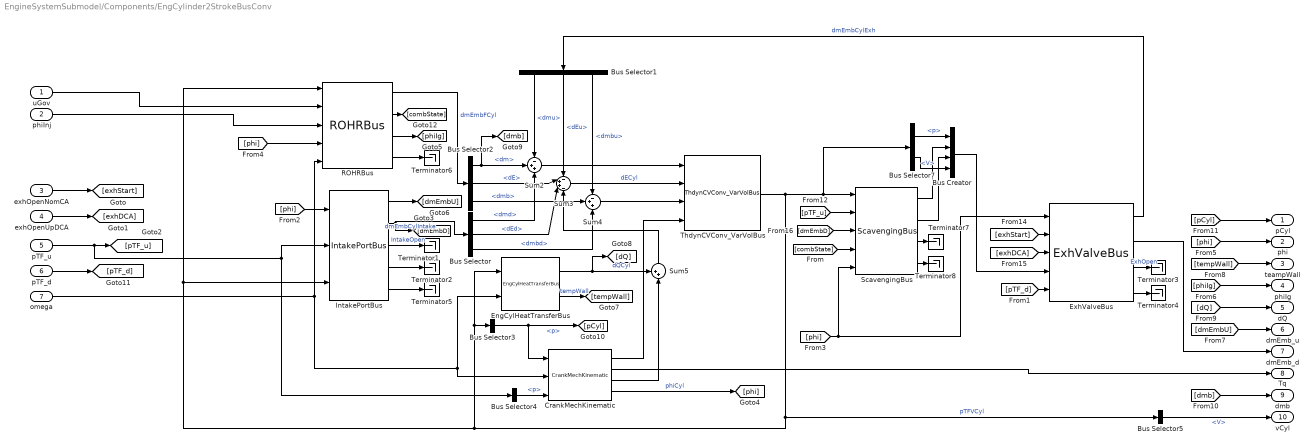
== system EngineSystemSubmodel/Components/EngCylinder2StrokeBusConv ==
  uGov : Inport
  phiInj : Inport  Port=2
  exhOpenNomCA : Inport  Port=3
  exhOpenUpDCA : Inport  Port=4
  pTF_u : Inport  Port=5
  pTF_d : Inport  Port=6
  omega : Inport  Port=7
  Bus Creator : BusCreator
  Bus Selector : BusSelector  OutputSignals=dmd,dEd,dmbd
  Bus Selector1 : BusSelector  OutputSignals=dmu,dEu,dmbu
  Bus Selector2 : BusSelector  OutputSignals=dm,dE,dmb
  Bus Selector3 : BusSelector  OutputSignals=p
  Bus Selector4 : BusSelector  OutputSignals=p
  Bus Selector5 : BusSelector  OutputSignals=V
  Bus Selector7 : BusSelector  OutputSignals=p,V
  CrankMechKinematic : EngineSystemSubmodel/Mechanical Part/CrankMechKinematic
  EngCylHeatTransferBus : EngineSystemSubmodel/Heat Transfer/EngCylHeatTransferBus
  ExhValveBus : EngineSystemSubmodel/Components/ExhValveBus
  IntakePortBus : EngineSystemSubmodel/Components/IntakePortBus
  ROHRBus : EngineSystemSubmodel/Combustion/ROHRBus
  ScavengingBus : EngineSystemSubmodel/Gas Exchange/ScavengingBus
  Sum2 : Sum  Inputs=-++
  Sum3 : Sum  Inputs=-++-
  Sum4 : Sum  Inputs=-++
  Sum5 : Sum  Inputs=++|
  Terminator{1..8} (8 alike) : Terminator
  ThdynCVConv_VarVolBus : EngineSystemSubmodel/Control Volume/ThdynCVConv_VarVolBus  CV=cyl.init
  pCyl : Outport
  phi : Outport  Port=2
  teampWall : Outport  Port=3
  phiIg : Outport  Port=4
  dQ : Outport  Port=5
  dmEmb_u : Outport  Port=6
  dmEmb_d : Outport  Port=7
  Tq : Outport  Port=8
  dmb : Outport  Port=9
  vCyl : Outport  Port=10
  wires:
  IntakePortBus/2 -> [dmEmbD], Bus Selector/1  "dmEmbCylIntake"
  Sum2/1 -> ThdynCVConv_VarVolBus/1
  Sum3/1 -> ThdynCVConv_VarVolBus/2  "dECyl"
  Sum4/1 -> ThdynCVConv_VarVolBus/3
  ExhValveBus/1 -> Bus Selector1/1  "dmEmbCylExh"
  Bus Selector1/1 -> Sum2/1  "<dmu>"
  Bus Selector1/2 -> Sum3/1  "<dEu>"
  Bus Selector1/3 -> Sum4/1  "<dmbu>"
  Bus Selector/1 -> Sum2/3  "<dmd>"
  ROHRBus/1 -> Bus Selector2/1  "dmEmbFCyl"
  Bus Selector2/1 -> [dmb], Sum2/2  "<dm>"
  Bus Selector/2 -> Sum3/3  "<dEd>"
  Bus Selector/3 -> Sum4/3  "<dmbd>"
  Bus Selector2/3 -> Sum4/2  "<dmb>"
  omega/1 -> ROHRBus/5, CrankMechKinematic/2, EngCylHeatTransferBus/2
  Bus Selector3/1 -> CrankMechKinematic/1, [pCyl]  "<p>"
  CrankMechKinematic/2 -> Tq/1
  CrankMechKinematic/1 -> ThdynCVConv_VarVolBus/4
  EngCylHeatTransferBus/1 -> [dQ], Sum5/1  "dQCyl"
  CrankMechKinematic/4 -> [phi]  "phiCyl"
  [phi] -> IntakePortBus/1
  [phi] -> ExhValveBus/1, ScavengingBus/5
  pTF_u/1 -> [pTF_u], IntakePortBus/2, Bus Selector4/1
  Bus Selector4/1 -> CrankMechKinematic/3  "<p>"
  exhOpenNomCA/1 -> [exhStart]
  exhOpenUpDCA/1 -> [exhDCA]
  [phi] -> ROHRBus/4
  ROHRBus/3 -> [phiIg]
  [phiIg] -> phiIg/1
  [phi] -> phi/1
  IntakePortBus/1 -> [dmEmbU]
  [dmEmbU] -> dmEmb_u/1
  ExhValveBus/2 -> dmEmb_d/1
  EngCylHeatTransferBus/2 -> [tempWall]  "tempWall"
  [tempWall] -> teampWall/1
  [dQ] -> dQ/1
  [dmb] -> dmb/1
  [pCyl] -> pCyl/1
  [exhStart] -> ExhValveBus/2
  [exhDCA] -> ExhValveBus/3
  ROHRBus/2 -> [combState]
  IntakePortBus/3 -> Terminator1/1  "IntakeOpen"
  IntakePortBus/4 -> Terminator2/1
  ExhValveBus/3 -> Terminator3/1  "ExhOpen"
  ExhValveBus/4 -> Terminator4/1
  Sum5/1 -> Sum3/4
  Bus Selector2/2 -> Sum3/2  "<dE>"
  uGov/1 -> ROHRBus/2
  phiInj/1 -> ROHRBus/3
  pTF_d/1 -> [pTF_d]
  [pTF_d] -> ExhValveBus/5
  CrankMechKinematic/3 -> Sum5/2
  IntakePortBus/5 -> Terminator5/1
  Bus Selector5/1 -> vCyl/1  "<V>"
  ROHRBus/4 -> Terminator6/1
  [pTF_u] -> ScavengingBus/2
  [dmEmbD] -> ScavengingBus/3
  [combState] -> ScavengingBus/4
  ScavengingBus/3 -> Terminator7/1
  ScavengingBus/4 -> Terminator8/1
  ThdynCVConv_VarVolBus/1 -> Bus Selector7/1, ScavengingBus/1, ROHRBus/1, IntakePortBus/3, EngCylHeatTransferBus/1, Bus Selector3/1, Bus Selector5/1  "pTFVCyl"
  Bus Selector7/1 -> Bus Creator/1  "<p>"
  Bus Creator/1 -> ExhValveBus/4
  ScavengingBus/1 -> Bus Creator/2
  ScavengingBus/2 -> Bus Creator/3
  Bus Selector7/2 -> Bus Creator/4  "<V>"

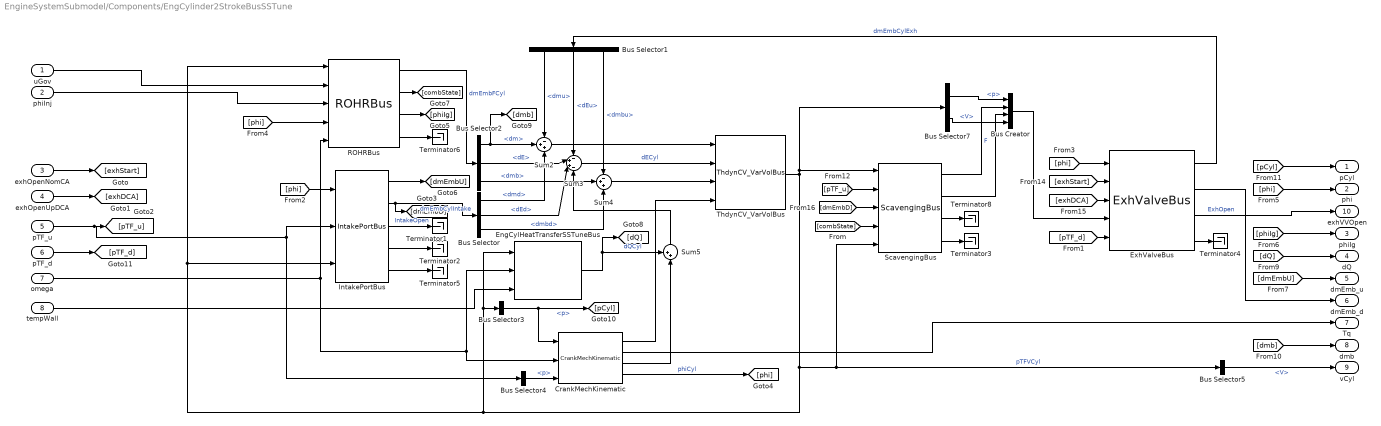
== system EngineSystemSubmodel/Components/EngCylinder2StrokeBusSSTune ==
  uGov : Inport
  phiInj : Inport  Port=2
  exhOpenNomCA : Inport  Port=3
  exhOpenUpDCA : Inport  Port=4
  pTF_u : Inport  Port=5
  pTF_d : Inport  Port=6
  omega : Inport  Port=7
  tempWall : Inport  Port=8
  Bus Creator : BusCreator
  Bus Selector : BusSelector  OutputSignals=dmd,dEd,dmbd
  Bus Selector1 : BusSelector  OutputSignals=dmu,dEu,dmbu
  Bus Selector2 : BusSelector  OutputSignals=dm,dE,dmb
  Bus Selector3 : BusSelector  OutputSignals=p
  Bus Selector4 : BusSelector  OutputSignals=p
  Bus Selector5 : BusSelector  OutputSignals=V
  Bus Selector7 : BusSelector  OutputSignals=p,V
  CrankMechKinematic : EngineSystemSubmodel/Mechanical Part/CrankMechKinematic
  EngCylHeatTransferSSTuneBus : EngineSystemSubmodel/Heat Transfer/EngCylHeatTransferSSTuneBus
  ExhValveBus : EngineSystemSubmodel/Components/ExhValveBus
  IntakePortBus : EngineSystemSubmodel/Components/IntakePortBus
  ROHRBus : EngineSystemSubmodel/Combustion/ROHRBus
  ScavengingBus : EngineSystemSubmodel/Gas Exchange/ScavengingBus
  Sum2 : Sum  Inputs=-++
  Sum3 : Sum  Inputs=-++-
  Sum4 : Sum  Inputs=-++
  Sum5 : Sum  Inputs=++|
  Terminator{1..6,8} (7 alike) : Terminator
  ThdynCV_VarVolBus : EngineSystemSubmodel/Control Volume/ThdynCV_VarVolBus  CV=cyl.init
  pCyl : Outport
  phi : Outport  Port=2
  phiIg : Outport  Port=3
  dQ : Outport  Port=4
  dmEmb_u : Outport  Port=5
  dmEmb_d : Outport  Port=6
  Tq : Outport  Port=7
  dmb : Outport  Port=8
  vCyl : Outport  Port=9
  exhVVOpen : Outport  Port=10
  wires:
  ROHRBus/4 -> Terminator6/1
  Bus Selector5/1 -> vCyl/1  "<V>"
  IntakePortBus/5 -> Terminator5/1
  CrankMechKinematic/3 -> Sum5/2
  [pTF_d] -> ExhValveBus/5
  pTF_d/1 -> [pTF_d]
  phiInj/1 -> ROHRBus/3
  uGov/1 -> ROHRBus/2
  Bus Selector2/2 -> Sum3/2  "<dE>"
  Sum5/1 -> Sum3/4
  ExhValveBus/4 -> Terminator4/1
  ExhValveBus/3 -> exhVVOpen/1  "ExhOpen"
  IntakePortBus/4 -> Terminator2/1
  IntakePortBus/3 -> Terminator1/1  "IntakeOpen"
  ROHRBus/2 -> [combState]
  [exhDCA] -> ExhValveBus/3
  [exhStart] -> ExhValveBus/2
  [pCyl] -> pCyl/1
  [dmb] -> dmb/1
  [dQ] -> dQ/1
  ExhValveBus/2 -> dmEmb_d/1
  [dmEmbU] -> dmEmb_u/1
  IntakePortBus/1 -> [dmEmbU]
  [phi] -> phi/1
  [phiIg] -> phiIg/1
  ROHRBus/3 -> [phiIg]
  [phi] -> ROHRBus/4
  exhOpenUpDCA/1 -> [exhDCA]
  exhOpenNomCA/1 -> [exhStart]
  Bus Selector4/1 -> CrankMechKinematic/3  "<p>"
  pTF_u/1 -> IntakePortBus/2, Bus Selector4/1, [pTF_u]
  [phi] -> IntakePortBus/1
  CrankMechKinematic/4 -> [phi]  "phiCyl"
  EngCylHeatTransferSSTuneBus/1 -> Sum5/1, [dQ]  "dQCyl"
  CrankMechKinematic/1 -> ThdynCV_VarVolBus/4
  CrankMechKinematic/2 -> Tq/1
  Bus Selector3/1 -> [pCyl], CrankMechKinematic/1  "<p>"
  omega/1 -> EngCylHeatTransferSSTuneBus/2, CrankMechKinematic/2, ROHRBus/5
  Bus Selector2/3 -> Sum4/2  "<dmb>"
  Bus Selector/3 -> Sum4/3  "<dmbd>"
  Bus Selector/2 -> Sum3/3  "<dEd>"
  Bus Selector2/1 -> Sum2/2, [dmb]  "<dm>"
  ROHRBus/1 -> Bus Selector2/1  "dmEmbFCyl"
  Bus Selector/1 -> Sum2/3  "<dmd>"
  Bus Selector1/3 -> Sum4/1  "<dmbu>"
  Bus Selector1/2 -> Sum3/1  "<dEu>"
  Bus Selector1/1 -> Sum2/1  "<dmu>"
  ExhValveBus/1 -> Bus Selector1/1  "dmEmbCylExh"
  Sum4/1 -> ThdynCV_VarVolBus/3
  Sum3/1 -> ThdynCV_VarVolBus/2  "dECyl"
  Sum2/1 -> ThdynCV_VarVolBus/1
  IntakePortBus/2 -> [dmEmbD], Bus Selector/1  "dmEmbCylIntake"
  tempWall/1 -> EngCylHeatTransferSSTuneBus/3
  [phi] -> ExhValveBus/1
  [pTF_u] -> ScavengingBus/2
  [combState] -> ScavengingBus/4
  ScavengingBus/3 -> Terminator8/1
  ThdynCV_VarVolBus/1 -> Bus Selector7/1, ScavengingBus/1, ScavengingBus/5, Bus Selector5/1, EngCylHeatTransferSSTuneBus/1, Bus Selector3/1, IntakePortBus/3, ROHRBus/1  "pTFVCyl"
  Bus Selector7/1 -> Bus Creator/1  "<p>"
  Bus Selector7/2 -> Bus Creator/4  "<V>"
  Bus Creator/1 -> ExhValveBus/4
  [dmEmbD] -> ScavengingBus/3
  ScavengingBus/1 -> Bus Creator/2  "F"
  ScavengingBus/2 -> Bus Creator/3
  ScavengingBus/4 -> Terminator3/1

== system EngineSystemSubmodel/Components/EngCylinder2StrokeConv ==
  uGov : Inport
  phiInj : Inport  Port=2
  cAStartNom : Inport  Port=3
  dCALiftUp : Inport  Port=4
  pTF_u : Inport  Port=5
  pTF_d : Inport  Port=6
  omega : Inport  Port=7
  Constant : Constant  Value=0
  CrankMechKinematic : EngineSystemSubmodel/Mechanical Part/CrankMechKinematic
  Demux{,1..3,5} (5 alike) : Demux  Outputs=3
  EngCylHeatTransfer : EngineSystemSubmodel/Heat Transfer/EngCylHeatTransfer
  ExhValve : EngineSystemSubmodel/Components/ExhValve
  IntakePort1 : EngineSystemSubmodel/Components/IntakePort
  Mux : Mux  Inputs=3
  Mux1 : Mux  Inputs=3
  Mux2 : Mux  Inputs=2
  Mux3 : Mux  Inputs=3
  ROHR1 : EngineSystemSubmodel/Combustion/ROHR
  Scavenging : EngineSystemSubmodel/Gas Exchange/Scavenging
  Sum : Sum  Inputs=++--
  Sum1 : Sum  Inputs=++|
  Terminator{1..3,6..9,11,13..14,16} (11 alike) : Terminator
  ThdynCVConv_VarVol : EngineSystemSubmodel/Control Volume/ThdynCVConv_VarVol  CV=cyl.init
  pCyl : Outport
  phi : Outport  Port=2
  teampWall : Outport  Port=3
  phiIg : Outport  Port=4
  dQ : Outport  Port=5
  dmEmb_u : Outport  Port=6
  dmEmb_d : Outport  Port=7
  Tq : Outport  Port=8
  dmb : Outport  Port=9
  wires:
  Mux3/1 -> ExhValve/4
  [cAStartNom] -> ExhValve/2
  dCALiftUp/1 -> [dCALiftUp]
  cAStartNom/1 -> [cAStartNom]
  ExhValve/2 -> dmEmb_d/1
  Mux2/1 -> Terminator2/1
  ExhValve/4 -> Mux2/2
  ExhValve/3 -> Mux2/1
  Mux1/1 -> Terminator1/1
  IntakePort1/5 -> Mux1/3
  IntakePort1/4 -> Mux1/2
  IntakePort1/3 -> Mux1/1
  ROHR1/3 -> phiIg/1  "phiIg"
  EngCylHeatTransfer/2 -> teampWall/1
  Demux/3 -> Terminator7/1
  Demux/2 -> Terminator6/1
  Constant/1 -> Mux/3, Mux/1
  Mux/1 -> Sum/4
  Sum1/1 -> Mux/2
  EngCylHeatTransfer/1 -> Sum1/1, dQ/1
  ThdynCVConv_VarVol/3 -> EngCylHeatTransfer/2  "vCyl"
  IntakePort1/1 -> dmEmb_u/1
  omega/1 -> ROHR1/5, EngCylHeatTransfer/3, CrankMechKinematic/2
  phiInj/1 -> ROHR1/3
  CrankMechKinematic/2 -> Tq/1
  Demux/1 -> CrankMechKinematic/3
  CrankMechKinematic/3 -> Sum1/2
  uGov/1 -> ROHR1/2
  CrankMechKinematic/1 -> ThdynCVConv_VarVol/2
  ThdynCVConv_VarVol/2 -> CrankMechKinematic/1, pCyl/1
  ThdynCVConv_VarVol/1 -> EngCylHeatTransfer/1, Demux2/1, IntakePort1/3, ROHR1/1  "pTFCyl"
  Sum/1 -> ThdynCVConv_VarVol/1
  ExhValve/1 -> Sum/3
  ROHR1/1 -> Sum/2, Demux1/1  "dmEmbComb"
  Demux1/1 -> dmb/1
  Demux1/2 -> Terminator8/1
  Demux1/3 -> Terminator9/1
  ROHR1/4 -> Terminator3/1
  pTF_u/1 -> [pTFIn], Demux/1, IntakePort1/2
  pTF_d/1 -> ExhValve/5
  ROHR1/2 -> [combState]
  [pTFIn] -> Demux3/1
  Demux3/1 -> Scavenging/4  "pIn"
  Demux3/2 -> Scavenging/5
  Demux3/3 -> Scavenging/6
  [mDotIn] -> Scavenging/7
  CrankMechKinematic/4 -> [phi], IntakePort1/1, phi/1, Scavenging/9, ExhValve/1
  IntakePort1/2 -> Demux5/1, Sum/1
  Demux5/2 -> Terminator11/1
  Demux5/3 -> Terminator16/1
  Demux5/1 -> [mDotIn]
  [combState] -> Scavenging/8
  [phi] -> ROHR1/4
  Scavenging/3 -> Terminator13/1
  Scavenging/4 -> Terminator14/1
  Demux2/2 -> Scavenging/2
  Demux2/1 -> Mux3/1, Scavenging/1
  Demux2/3 -> Scavenging/3
  Scavenging/1 -> Mux3/2  "TOut"
  Scavenging/2 -> Mux3/3  "FOut"
  [dCALiftUp] -> ExhValve/3

== system EngineSystemSubmodel/Components/EngCylinder2StrokeSSTune ==
  uGov : Inport
  phiInj : Inport  Port=2
  cAStartNom : Inport  Port=3
  dCALiftUp : Inport  Port=4
  tWall : Inport  Port=5
  pTF_u : Inport  Port=6
  pTF_d : Inport  Port=7
  omega : Inport  Port=8
  Constant : Constant  Value=0
  CrankMechKinematic : EngineSystemSubmodel/Mechanical Part/CrankMechKinematic
  Demux{,1..3,5} (5 alike) : Demux  Outputs=3
  EngCylHeatTransferSSTune : EngineSystemSubmodel/Heat Transfer/EngCylHeatTransferSSTune
  ExhValve : EngineSystemSubmodel/Components/ExhValve
  IntakePort1 : EngineSystemSubmodel/Components/IntakePort
  Mux : Mux  Inputs=3
  Mux1 : Mux  Inputs=3
  Mux2 : Mux  Inputs=2
  Mux3 : Mux  Inputs=3
  ROHR1 : EngineSystemSubmodel/Combustion/ROHR
  Scavenging : EngineSystemSubmodel/Gas Exchange/Scavenging
  Sum : Sum  Inputs=++--
  Sum1 : Sum  Inputs=++|
  Terminator{1..3,6..9,11,13..14,16} (11 alike) : Terminator
  ThdynCV_VarVol1 : EngineSystemSubmodel/Control Volume/ThdynCV_VarVol  CV=cyl.init
  pCyl : Outport
  phi : Outport  Port=2
  phiIg : Outport  Port=3
  dQ : Outport  Port=4
  dmEmb_u : Outport  Port=5
  dmEmb_d : Outport  Port=6
  Tq : Outport  Port=7
  dmb : Outport  Port=8
  wires:
  [dCALiftUp] -> ExhValve/3
  Scavenging/2 -> Mux3/3  "FOut"
  Scavenging/1 -> Mux3/2  "TOut"
  Demux2/3 -> Scavenging/3
  Demux2/1 -> Scavenging/1, Mux3/1
  Demux2/2 -> Scavenging/2
  Scavenging/4 -> Terminator14/1
  Scavenging/3 -> Terminator13/1
  [phi] -> ROHR1/4
  [combState] -> Scavenging/8
  Demux5/1 -> [mDotIn]
  Demux5/3 -> Terminator16/1
  Demux5/2 -> Terminator11/1
  IntakePort1/2 -> Sum/1, Demux5/1
  CrankMechKinematic/4 -> ExhValve/1, Scavenging/9, phi/1, IntakePort1/1, [phi]
  [mDotIn] -> Scavenging/7
  Demux3/3 -> Scavenging/6
  Demux3/2 -> Scavenging/5
  Demux3/1 -> Scavenging/4  "pIn"
  [pTFIn] -> Demux3/1
  ROHR1/2 -> [combState]
  pTF_d/1 -> ExhValve/5
  pTF_u/1 -> IntakePort1/2, Demux/1, [pTFIn]
  ROHR1/4 -> Terminator3/1
  Demux1/3 -> Terminator9/1
  Demux1/2 -> Terminator8/1
  Demux1/1 -> dmb/1
  ROHR1/1 -> Demux1/1, Sum/2  "dmEmbComb"
  ExhValve/1 -> Sum/3
  Sum/1 -> ThdynCV_VarVol1/1
  ThdynCV_VarVol1/1 -> ROHR1/1, IntakePort1/3, EngCylHeatTransferSSTune/1, Demux2/1  "pTFCyl"
  ThdynCV_VarVol1/2 -> pCyl/1, CrankMechKinematic/1
  CrankMechKinematic/1 -> ThdynCV_VarVol1/2
  uGov/1 -> ROHR1/2
  CrankMechKinematic/3 -> Sum1/2
  Demux/1 -> CrankMechKinematic/3
  CrankMechKinematic/2 -> Tq/1
  phiInj/1 -> ROHR1/3
  omega/1 -> EngCylHeatTransferSSTune/3, CrankMechKinematic/2, ROHR1/5
  IntakePort1/1 -> dmEmb_u/1
  ThdynCV_VarVol1/3 -> EngCylHeatTransferSSTune/2  "vCyl"
  EngCylHeatTransferSSTune/1 -> dQ/1, Sum1/1
  Sum1/1 -> Mux/2
  Mux/1 -> Sum/4
  Constant/1 -> Mux/1, Mux/3
  Demux/2 -> Terminator6/1
  Demux/3 -> Terminator7/1
  ROHR1/3 -> phiIg/1  "phiIg"
  IntakePort1/3 -> Mux1/1
  IntakePort1/4 -> Mux1/2
  IntakePort1/5 -> Mux1/3
  Mux1/1 -> Terminator1/1
  ExhValve/3 -> Mux2/1
  ExhValve/4 -> Mux2/2
  Mux2/1 -> Terminator2/1
  ExhValve/2 -> dmEmb_d/1
  cAStartNom/1 -> [cAStartNom]
  dCALiftUp/1 -> [dCALiftUp]
  [cAStartNom] -> ExhValve/2
  Mux3/1 -> ExhValve/4
  tWall/1 -> [tWall]
  [tWall] -> EngCylHeatTransferSSTune/4

== system EngineSystemSubmodel/Components/EngCylinder2StrokeSSTune_ExtendedOutput ==
  uGov : Inport
  phiInj : Inport  Port=2
  cAStartNom : Inport  Port=3
  dCALiftUp : Inport  Port=4
  tempWall : Inport  Port=5
  pTF_u : Inport  Port=6
  pTF_d : Inport  Port=7
  omega : Inport  Port=8
  Constant : Constant  Value=0
  CrankMechKinematic : EngineSystemSubmodel/Mechanical Part/CrankMechKinematic
  Demux{,1..3,5} (5 alike) : Demux  Outputs=3
  EngCylHeatTransferSSTune : EngineSystemSubmodel/Heat Transfer/EngCylHeatTransferSSTune
  ExhValve : EngineSystemSubmodel/Components/ExhValve
  IntakePort1 : EngineSystemSubmodel/Components/IntakePort
  Mux : Mux  Inputs=3
  Mux1 : Mux  Inputs=3
  Mux3 : Mux  Inputs=3
  ROHR1 : EngineSystemSubmodel/Combustion/ROHR
  Scavenging : EngineSystemSubmodel/Gas Exchange/Scavenging
  Sum : Sum  Inputs=++--
  Sum1 : Sum  Inputs=++|
  Terminator{,1,3,6..9,11,13..14,16} (11 alike) : Terminator
  ThdynCV_VarVol1 : EngineSystemSubmodel/Control Volume/ThdynCV_VarVol  CV=cyl.init
  pCyl : Outport
  phi : Outport  Port=2
  phiIg : Outport  Port=3
  dQ : Outport  Port=4
  dmEmb_u : Outport  Port=5
  dmEmb_d : Outport  Port=6
  Tq : Outport  Port=7
  exhVVAOpen : Outport  Port=8
  vCyl : Outport  Port=9
  dmb : Outport  Port=10
  wires:
  [dCALiftUp] -> ExhValve/3
  Scavenging/2 -> Mux3/3  "FOut"
  Scavenging/1 -> Mux3/2  "TOut"
  Demux2/3 -> Scavenging/3
  Demux2/1 -> Scavenging/1, Mux3/1
  Demux2/2 -> Scavenging/2
  Scavenging/4 -> Terminator14/1
  Scavenging/3 -> Terminator13/1
  [phi] -> ROHR1/4
  [combState] -> Scavenging/8
  Demux5/1 -> [mDotIn]
  Demux5/3 -> Terminator16/1
  Demux5/2 -> Terminator11/1
  IntakePort1/2 -> Sum/1, Demux5/1
  CrankMechKinematic/4 -> ExhValve/1, Scavenging/9, phi/1, IntakePort1/1, [phi]
  [mDotIn] -> Scavenging/7
  Demux3/3 -> Scavenging/6
  Demux3/2 -> Scavenging/5
  Demux3/1 -> Scavenging/4  "pIn"
  [pTFIn] -> Demux3/1
  ROHR1/2 -> [combState]
  pTF_d/1 -> ExhValve/5
  pTF_u/1 -> IntakePort1/2, Demux/1, [pTFIn]
  ROHR1/4 -> Terminator3/1
  Demux1/3 -> Terminator9/1
  Demux1/2 -> Terminator8/1
  Demux1/1 -> dmb/1
  ROHR1/1 -> Demux1/1, Sum/2  "dmEmbComb"
  ExhValve/1 -> Sum/3
  Sum/1 -> ThdynCV_VarVol1/1
  ThdynCV_VarVol1/1 -> ROHR1/1, IntakePort1/3, EngCylHeatTransferSSTune/1, Demux2/1  "pTFCyl"
  ThdynCV_VarVol1/2 -> pCyl/1, CrankMechKinematic/1
  CrankMechKinematic/1 -> ThdynCV_VarVol1/2
  uGov/1 -> ROHR1/2
  CrankMechKinematic/3 -> Sum1/2
  Demux/1 -> CrankMechKinematic/3
  CrankMechKinematic/2 -> Tq/1
  phiInj/1 -> ROHR1/3
  omega/1 -> EngCylHeatTransferSSTune/3, CrankMechKinematic/2, ROHR1/5
  IntakePort1/1 -> dmEmb_u/1
  ThdynCV_VarVol1/3 -> EngCylHeatTransferSSTune/2, vCyl/1  "vCyl"
  EngCylHeatTransferSSTune/1 -> Sum1/1, dQ/1
  Sum1/1 -> Mux/2
  Mux/1 -> Sum/4
  Constant/1 -> Mux/1, Mux/3
  Demux/2 -> Terminator6/1
  Demux/3 -> Terminator7/1
  ROHR1/3 -> phiIg/1  "phiIg"
  IntakePort1/3 -> Mux1/1
  IntakePort1/4 -> Mux1/2
  IntakePort1/5 -> Mux1/3
  Mux1/1 -> Terminator1/1
  ExhValve/3 -> exhVVAOpen/1
  ExhValve/4 -> Terminator/1
  ExhValve/2 -> dmEmb_d/1
  cAStartNom/1 -> [cAStartNom]
  dCALiftUp/1 -> [dCALiftUp]
  [cAStartNom] -> ExhValve/2
  Mux3/1 -> ExhValve/4  "pTFCylOut"
  tempWall/1 -> [tempWall]
  [tempWall] -> EngCylHeatTransferSSTune/4
